simulink model "Obs2_simulink"  (R2021a)
settings: Solver=VariableStepAuto  StartTime=0.0  StopTime=Inf  RelTol=1e-3
values from neighbouring files (symbols this model uses):
  A_d = I + A*Ts    [observador_completo.m]
  C_d = C    [observador_completo.m]
  L = place(A_d', C_d', p_obs_d)'    [observador_completo.m]
libraries: instrumentseriallib x2
settings Model: Creator=Claudio  LastModifiedBy=mogic

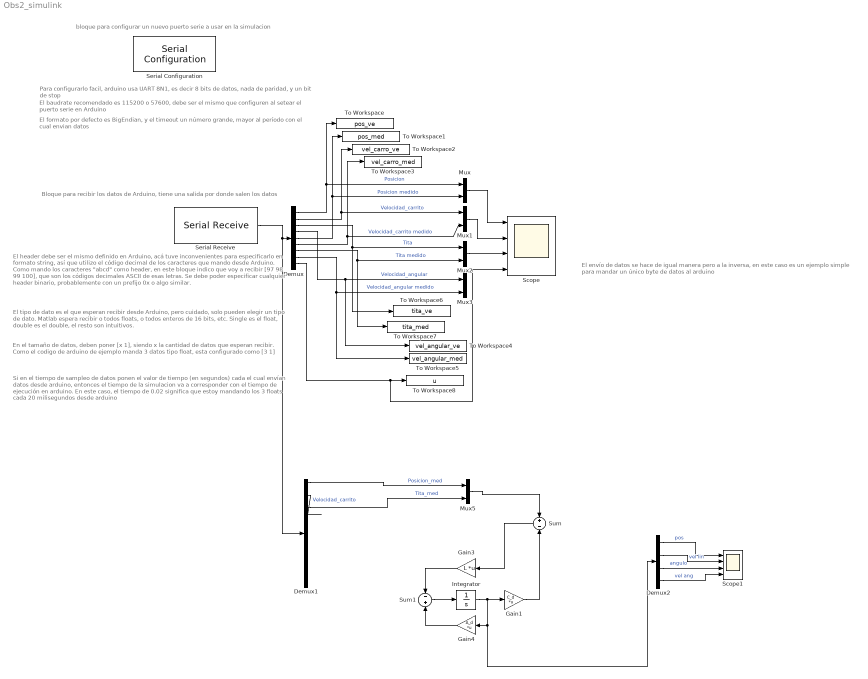
== system Obs2_simulink ==
  note: El envío de datos se hace de igual manera pero a la inversa, en este caso es un ejemplo simple para mandar un único byte de datos al arduino
  note: Si en el tiempo de sampleo de datos ponen el valor de tiempo (en segundos) cada el cual envían datos desde arduino, entonces el tiempo de la simulacion va a corresponder con el tiempo de ejecución en arduino. En este caso, el tiempo de 0.02 significa que estoy mandando los 3 floats cada 20 milisegundos desde arduino
  note: En el tamaño de datos, deben poner [x 1], siendo x la cantidad de datos que esperan recibir. Como el codigo de arduino de ejemplo manda 3 datos tipo float, esta configurado como [3 1]
  note: El tipo de dato es el que esperan recibir desde Arduino, pero cuidado, solo pueden elegir un tipo de dato. Matlab espera recibir o todos floats, o todos enteros de 16 bits, etc. Single es el float, double es el double, el resto son intuitivos.
  note: El header debe ser el mismo definido en Arduino, acá tuve inconvenientes para especificarlo en formato string, así que utilizo el código decimal de los caracteres que mando desde Arduino. Como mando los caracteres "abcd" como header, en este bloque indico que voy a recibir [97 98 99 100], que son los códigos decimales ASCII de esas letras. Se debe poder especificar cualquier header binario, probablemente con un prefijo 0x o algo similar.
  note: Bloque para recibir los datos de Arduino, tiene una salida por donde salen los datos
  note: El formato por defecto es BigEndian, y el timeout un número grande, mayor al período con el cual envian datos
  note: El baudrate recomendado es 115200 o 57600, debe ser el mismo que configuren al setear el puerto serie en Arduino
  note: Para configurarlo facil, arduino usa UART 8N1, es decir 8 bits de datos, nada de paridad, y un bit de stop
  note: bloque para configurar un nuevo puerto serie a usar en la simulacion
  Demux : Demux  Outputs=9
  Demux1 : Demux  Outputs=9
  Demux2 : Demux
  Gain1 : Gain  Gain=C_d  Multiplication=Matrix(K*u)
  Gain3 : Gain  Gain=L  Multiplication=Matrix(K*u)
  Gain4 : Gain  Gain=A_d  Multiplication=Matrix(K*u)
  Integrator : Integrator
  Mux{,1..3,5} (5 alike) : Mux  Inputs=2
  Scope : Scope  NumInputPorts=4
  Scope1 : Scope  NumInputPorts=4
  Serial Configuration : instrumentseriallib/Serial Configuration  Priority=-200000  Port=COM3  ComPort=COM3  BaudRate=115200  DataBits=8  Parity=none  StopBits=1  ByteOrder=big-endian  FlowControl=none  Timeout=10  SimulateUsing=Interpreted execution  BlockInModel=on
  Serial Receive : instrumentseriallib/Serial Receive  Priority=1  Port=COM3  ComPort=COM3  DataType=single  SaveDataType=uint8  ToggleHeader=on  Header="[ 97   98   99  100 ]"  ToggleTerminator=off  Terminator=<none>  CustomTerminator=[]  ToggleDataSize=on  DataSize=[9 1]  EnableBlockingMode=on  ActionDataUnavailable=Output last received value  ActionWhenDataUnavailable=Output last received value  CustomValue=0  SampleTime=0.02  SimulateUsing=Interpreted execution  BlockInModel=on
  Sum : Sum  Inputs=+|-
  Sum1 : Sum  Inputs=-+
  To Workspace : ToWorkspace  VariableName=pos_ve  SampleTime=-1
      settings: Save2DSignal=2-D array (concatenate along first dimension)
  To Workspace1 : ToWorkspace  VariableName=pos_med  SampleTime=-1
      settings: Save2DSignal=2-D array (concatenate along first dimension)
  To Workspace2 : ToWorkspace  VariableName=vel_carro_ve  SampleTime=-1
      settings: Save2DSignal=2-D array (concatenate along first dimension)
  To Workspace3 : ToWorkspace  VariableName=vel_carro_med  SampleTime=-1
      settings: Save2DSignal=2-D array (concatenate along first dimension)
  To Workspace4 : ToWorkspace  VariableName=vel_angular_ve  SampleTime=-1
      settings: Save2DSignal=2-D array (concatenate along first dimension)
  To Workspace5 : ToWorkspace  VariableName=vel_angular_med  SampleTime=-1
      settings: Save2DSignal=2-D array (concatenate along first dimension)
  To Workspace6 : ToWorkspace  VariableName=tita_ve  SampleTime=-1
      settings: Save2DSignal=2-D array (concatenate along first dimension)
  To Workspace7 : ToWorkspace  VariableName=tita_med  SampleTime=-1
      settings: Save2DSignal=2-D array (concatenate along first dimension)
  To Workspace8 : ToWorkspace  VariableName=u  SampleTime=-1
      settings: Save2DSignal=2-D array (concatenate along first dimension)
  wires:
  Demux/2 -> To Workspace2/1, Mux1/1  "Velocidad_carrito"
  Demux/1 -> To Workspace/1, Mux/1  "Posicion"
  Serial Receive/1 -> Demux1/1, Demux/1
  Demux/3 -> To Workspace6/1, Mux2/1  "Tita"
  Demux/4 -> To Workspace4/1, Mux3/1  "Velocidad_angular"
  Mux/1 -> Scope/1
  Demux/5 -> To Workspace1/1, Mux/2  "Posicion medido"
  Demux/6 -> To Workspace3/1, Mux1/2  "Velocidad_carrito medido"
  Demux/7 -> To Workspace7/1, Mux2/2  "Tita medido"
  Demux/8 -> To Workspace5/1, Mux3/2  "Velocidad_angular medido"
  Mux1/1 -> Scope/2
  Mux2/1 -> Scope/3
  Demux/9 -> Scope/4, To Workspace8/1
  Demux1/1 -> Mux5/1  "Posicion_med"
  Demux1/2 -> ?  "Velocidad_carrito"
  Demux2/2 -> Scope1/2  "vel lin"
  Demux2/4 -> Scope1/4  "vel ang"
  Demux2/3 -> Scope1/3  "angulo"
  Demux2/1 -> Scope1/1  "pos"
  Demux1/3 -> Mux5/2  "Tita_med"
  Mux5/1 -> Sum/1
  Gain1/1 -> Sum/2
  Sum/1 -> Gain3/1
  Sum1/1 -> Integrator/1
  Integrator/1 -> Demux2/1, Gain4/1, Gain1/1
  Gain3/1 -> Sum1/1
  Gain4/1 -> Sum1/2
